simulink model "Chapter_4_Section_3_Model"  (R2017a)
settings: Solver=ode4  StartTime=0.0  StopTime=200  FixedStep=stp_sz  MaxStep=.0001  MinStep=.00005  RelTol=1e-7  AbsTol=1e-7  EnableMultiTasking=on
InitFcn:
  | load Chapter_4_Section_3
  | warning off
StopFcn:
  | save data.mat u_simulation v_simulation psi_simulation r_simulation npr_user_provided npr_achievable alpha_user_provided alpha_achievable stp_sz
  | clear all
  | load('data.mat')
  | delete('data.mat')
values from neighbouring files (symbols this model uses):
  A_disk = 13.2025431267    [Chapter_4_Section_3.mat]
  a_r11 = [-0.000865667853776 -0.901318756108 0.00874486630837 -0.00765974060328 0.00955717632387 0.00641813989061 -0.011076069832 0.00201248118094 -0.00501952733262 0.00315605586996 -0.00210851076531 0.0148609220099 ... (324 elements, 18x18)]    [Chapter_4_Section_3.mat]
  a_r13 = [-0.0294995912119 -4.91037219533 -0.00332739568397 0.0888755061346 -0.00681796875441 0.183812407485 0.0112008036726 0.10429312155 -0.0251601482875 -0.228675692165 0.00453476042855 0.0594697753606 ... (169 elements, 13x13)]    [Chapter_4_Section_3.mat]
  a_r15 = [-0.00127786555898 0.776225741104 -0.00474776997752 -0.00131066749835 0.0137520402687 -0.00211384579247 8.8019955143e-05 -0.00028996241197 -0.00129826872567 -0.0202543144732 0.0030370404199 -0.00453425604591 ... (169 elements, 13x13)]    [Chapter_4_Section_3.mat]
  a_r22 = [-0.000797108949019 -1.01015556887 0.00406573750109 -0.00111578544774 0.00423859757219 -0.00799128279013 0.00569024815652 -0.0167562674532 0.00334935655618 -0.000712432292804 0.00154242142086 0.00240437743229 ... (169 elements, 13x13)]    [Chapter_4_Section_3.mat]
  a_r24 = [-0.000686927823555 -0.95665602689 0.00244839898375 0.00145613314595 -0.00607023426216 0.0163996841317 0.00152022458075 -0.000736874734971 -0.00294919321651 -0.000761800577268 -0.00251686123035 -0.00197732815976 ... (169 elements, 13x13)]    [Chapter_4_Section_3.mat]
  a_r26 = [-0.194397873228 1.89810259721 -0.0873186628061 -0.241231729519 0.281206161775 -0.16994038615 -0.116565511469 -0.0496572593209 0.0216084469732 0.0912933167406 0.0299797727001 0.0314987707028 ... (169 elements, 13x13)]    [Chapter_4_Section_3.mat]
  a_r31 = [-0.00489112559449 -3.89960530455 -0.0361162658575 0.0265931197764 0.0034376033088 0.000316401308368 -0.0243996243526 0.0792200139858 -0.023187698537 -0.0726743997029 0.00400632061963 -0.0350516560041 ... (169 elements, 13x13)]    [Chapter_4_Section_3.mat]
  a_r33 = [-0.601431448276 0.50360246711 0.500115950342 -0.0452293844892 -0.0181314142185 -0.0323524621531 0.0355826051968 0.0329239610677 0.0940919952313 0.0566642992805 -0.0379178935102 0.0254835488846 ... (169 elements, 13x13)]    [Chapter_4_Section_3.mat]
  a_r35 = [-0.861988746714 -0.582511154549 0.34264856173 -0.0655310417272 -0.417167685168 0.183176698588 -0.473887691644 -0.225677727522 -0.133571139717 -0.218168843707 0.0850592077583 -0.0257492082836 ... (169 elements, 13x13)]    [Chapter_4_Section_3.mat]
  a_r42 = [-0.000411079312172 -0.966350953459 0.00419936729713 0.00358740198521 -0.00356571428733 -0.00958951498266 -0.00230062261745 -3.48708248632e-05 -0.00350313209064 -0.00772126326768 -0.0011918234528 -0.00149424537901 ... (169 elements, 13x13)]    [Chapter_4_Section_3.mat]
  a_r44 = [-0.000156115728087 -0.944139704333 -0.00242185567679 0.00620214191605 0.00232565005277 -0.00625050722164 0.00126021167241 -0.000681873506535 0.0011931592381 -0.00289361611357 -0.00138182415247 -0.00252837386868 ... (169 elements, 13x13)]    [Chapter_4_Section_3.mat]
  a_r46 = [-0.000218462457517 1.89677852742 0.00896242354968 -0.00290259500747 0.00225128874867 0.00254539590487 0.00120681433209 0.00261900930035 0.00149629742842 0.000796832004109 0.00199591847947 0.00352664402036 ... (169 elements, 13x13)]    [Chapter_4_Section_3.mat]
  a_r51 = [-0.0010898880101 0.776080724329 0.000225388678941 0.00375234840616 -0.00838297691459 -0.00447310416982 -0.0119510882322 -0.00692765468718 0.00227273345413 -0.0063592610709 0.000914007544175 0.00943534814934 ... (169 elements, 13x13)]    [Chapter_4_Section_3.mat]
  a_r53 = [-0.83377539904 0.569677058563 0.434285019976 0.157205409215 -0.397195569542 -0.255164078245 -0.141246880777 0.177451291189 -0.182828550566 0.0648162508754 0.244251292681 0.160100487197 ... (169 elements, 13x13)]    [Chapter_4_Section_3.mat]
  a_r55 = [-0.000352406331634 0.764343029796 0.00339830320259 -0.000678251137483 -0.00243783779313 -0.00215979913278 0.00196909451093 -0.00577428819561 -0.00349811892924 -0.00488920883323 0.00112064970343 0.000774855197444 ... (169 elements, 13x13)]    [Chapter_4_Section_3.mat]
  a_r62 = [-0.546519039316 -1.22303009993 0.393735845548 -0.120016588191 0.38151861373 -0.213578592342 -0.602267954372 -0.105716444149 -0.153151371839 -0.163939447448 -0.555540353196 0.0685401630267 ... (169 elements, 13x13)]    [Chapter_4_Section_3.mat]
  a_r64 = [-0.0406191100017 -5.18251105957 -0.115497941507 -0.0935821370219 0.180972853448 -0.0201998949456 -0.0698170640352 -0.0736823539521 -0.034828919888 0.0876659960431 -0.0419335596239 -0.0240984963396 ... (169 elements, 13x13)]    [Chapter_4_Section_3.mat]
  a_r66 = [-0.00276803466684 1.11530008029 0.0229779449181 0.0262185319857 0.00628472844795 0.000156167369042 -0.00250093023805 -0.0114435042874 -0.00826774415326 -0.00991601759993 -0.00812142854996 0.0148245002111 ... (169 elements, 13x13)]    [Chapter_4_Section_3.mat]
  A_rudder = 6    [Chapter_4_Section_3.mat]
  alpha_max = 0.392699081699    [Chapter_4_Section_3.mat]
  b_r11 = [-1.91804272115 -67.7547902158 12.3212653748 -6.25011871643 13.082442224 5.48501776184 -10.1596546398 2.56004852009 -4.74360113798 3.95981895348 -2.02856412397 18.3264246889 ... (18 elements, 18x1)]    [Chapter_4_Section_3.mat]
  b_r13 = [9.68113335046 8.54720242819 0.883931047444 -5.56576078332 1.72641800243 -13.8756826027 -2.702777864 -9.4621991361 5.92943514782 22.6516835054 -1.0074598861 -6.31102592982 ... (13 elements, 13x1)]    [Chapter_4_Section_3.mat]
  b_r22 = [-8.230214728 -263.156134326 24.2327808151 -4.87921448873 19.1715641288 -45.8768653263 26.6325387064 -91.9399975548 16.6663243552 -3.80929112747 7.68030110892 12.8381492859 ... (13 elements, 13x1)]    [Chapter_4_Section_3.mat]
  b_r24 = [20.6689502907 674.321335078 -41.3637763247 -19.2444203625 82.0775505272 -259.897803047 -22.2545830602 11.3827604156 43.2189922355 11.7516897475 36.9394390446 30.4503929007 ... (13 elements, 13x1)]    [Chapter_4_Section_3.mat]
  b_r26 = [206.794755218 -62.242559329 24.5666904254 184.158146246 -103.419961827 115.160111337 76.4499795128 20.3457431208 -13.1704465249 -41.5730935141 -18.1334448714 -14.4641153742 ... (13 elements, 13x1)]    [Chapter_4_Section_3.mat]
  b_r31 = [3.76230189948 5.16928151238 2.64945725635 -18.4251953385 -2.0625905672 -0.18887543415 4.20433084471 -14.07893046 13.0563354882 16.4007691754 -2.13849071942 8.28528512456 ... (13 elements, 13x1)]    [Chapter_4_Section_3.mat]
  b_r33 = [-425.265727934 16.4952177922 163.76327445 -15.539902078 -6.59006558263 -11.1862310226 12.8543123126 11.4260264426 33.8206936715 19.7626944669 -13.5783728882 8.91023495161 ... (13 elements, 13x1)]    [Chapter_4_Section_3.mat]
  b_r35 = [955.467057384 23.8174564739 -126.402446683 48.3788727465 168.435579445 -128.161344325 216.24493699 142.979450788 65.1193355403 134.911935543 -50.7648858119 13.1799100865 ... (13 elements, 13x1)]    [Chapter_4_Section_3.mat]
  b_r42 = [15.9360311823 665.959154186 -98.5777560157 -55.5400651809 61.9220987195 200.312325561 47.5124103398 0.631683490985 64.1219861023 155.750535985 22.3985447876 29.803792586 ... (13 elements, 13x1)]    [Chapter_4_Section_3.mat]
  b_r44 = [-27.1891200017 -1761.50772747 -283.391471232 367.311489951 182.522124626 -579.755911925 104.353356772 -62.2376848714 99.3185259533 -260.784153955 -116.536414334 -226.454300618 ... (13 elements, 13x1)]    [Chapter_4_Section_3.mat]
  b_r46 = [-26.6906838426 431.487773123 657.709356633 -144.976364483 114.646575538 180.775978583 85.0953284375 135.592940904 78.9082960716 55.2973047721 106.740201988 241.432567993 ... (13 elements, 13x1)]    [Chapter_4_Section_3.mat]
  b_r51 = [-27.9768378982 741.05041888 2.33758926296 57.3995096963 -127.005620965 -47.2947833409 -133.876425682 -98.5907202753 26.0445243962 -88.3721242204 10.7680008324 130.122749963 ... (13 elements, 13x1)]    [Chapter_4_Section_3.mat]
  b_r53 = [949.455593416 -23.2452293814 -157.318364745 -121.412853107 173.067821874 177.10214052 64.7164189373 -120.452255472 86.0623964314 -43.0643550932 -116.39314584 -105.497696438 ... (13 elements, 13x1)]    [Chapter_4_Section_3.mat]
  b_r55 = [-217.127382907 9506.32343029 1148.82922273 -188.742556573 -694.43970838 -709.996440288 566.872400877 -1877.38940059 -1026.37679575 -1566.80129668 332.089563592 247.692614281 ... (13 elements, 13x1)]    [Chapter_4_Section_3.mat]
  b_r62 = [259.61149635 16.5485296799 -38.0095496792 45.1883806678 -40.3107166739 78.3455844965 73.5107367495 37.0054960802 51.6709447748 22.7410486275 84.4875008959 -21.9559289205 ... (13 elements, 13x1)]    [Chapter_4_Section_3.mat]
  b_r64 = [156.539833252 187.686482031 376.820920142 59.4312894666 -548.902692032 17.0176436095 70.7484878223 206.821047291 37.1716677759 -243.032149857 114.824775027 27.0037475025 ... (13 elements, 13x1)]    [Chapter_4_Section_3.mat]
  b_r66 = [-314.266256408 5285.46587095 1093.01941502 1627.30071258 387.633965073 8.0986510694 -130.443621448 -701.343286032 -436.49966457 -600.0481003 -433.735518303 884.367320612 ... (13 elements, 13x1)]    [Chapter_4_Section_3.mat]
  bettas_CQ = [0 5.39 17.77 34.97 50.79 58.7 64.55 68.33 73.49 85.2 93.11 102.75 ... (40 elements, 1x40)]    [Chapter_4_Section_3.mat]    (also in looking_up_n.m = [0 5.39 17.77 34.97 50.79 58.7 64.55 68.33 73.49 85.2 93.11 )
  bettas_CT = [0 5.37 16.73 33.6 44.63 60.82 73.22 80.46 86.3 92.15 100.41 110.74 ... (52 elements, 1x52)]    [Chapter_4_Section_3.mat]    (also in looking_up_n.m = [0 5.37 16.73 33.6 44.63 60.82 73.22 80.46 86.3 92.15 100.41)
  c_r11 = [1.91804272142 -67.7547902158 -12.3212653748 -6.25011871643 -13.082442224 5.48501776185 -10.1596546398 -2.56004852009 -4.74360113798 -3.95981895348 -2.02856412396 -18.3264246889 ... (18 elements, 1x18)]    [Chapter_4_Section_3.mat]
  c_r13 = [9.68113335045 -8.54720242824 0.883931047418 5.56576078332 1.72641800244 13.8756826027 -2.702777864 9.4621991361 5.92943514781 -22.6516835054 -1.0074598861 6.31102592982 ... (13 elements, 1x13)]    [Chapter_4_Section_3.mat]
  c_r22 = [8.23021472807 -263.156134326 -24.2327808151 -4.87921448871 19.1715641288 45.8768653263 26.6325387064 91.9399975548 16.6663243552 3.80929112749 7.68030110892 -12.8381492859 ... (13 elements, 1x13)]    [Chapter_4_Section_3.mat]
  c_r24 = [20.6689502903 -674.321335078 -41.3637763247 19.2444203625 -82.0775505271 -259.897803047 22.2545830602 11.3827604156 -43.2189922355 11.7516897475 -36.9394390446 30.4503929007 ... (13 elements, 1x13)]    [Chapter_4_Section_3.mat]
  c_r26 = [-206.794755218 -62.2425593289 24.5666904254 -184.158146246 -103.419961827 -115.160111337 -76.4499795128 20.3457431209 13.1704465249 -41.5730935141 18.1334448714 -14.4641153742 ... (13 elements, 1x13)]    [Chapter_4_Section_3.mat]
  c_r31 = [3.76230189951 -5.16928151238 -2.64945725636 -18.4251953385 -2.0625905672 -0.188875434257 -4.2043308447 14.07893046 13.0563354882 -16.4007691754 -2.13849071943 -8.28528512456 ... (13 elements, 1x13)]    [Chapter_4_Section_3.mat]
  c_r33 = [-425.265727934 -16.4952177923 -163.76327445 15.539902078 -6.5900655826 11.1862310226 12.8543123126 -11.4260264426 33.8206936715 -19.7626944669 -13.5783728882 -8.91023495161 ... (13 elements, 1x13)]    [Chapter_4_Section_3.mat]
  c_r35 = [-955.467057384 23.8174564746 -126.402446683 -48.3788727464 168.435579445 128.161344325 216.24493699 -142.979450788 65.1193355403 -134.911935543 50.7648858119 13.1799100865 ... (13 elements, 1x13)]    [Chapter_4_Section_3.mat]
  c_r42 = [15.9360311824 -665.959154186 -98.5777560157 55.5400651809 -61.9220987195 200.312325561 47.5124103398 -0.631683490192 -64.1219861023 155.750535985 -22.3985447876 29.803792586 ... (13 elements, 1x13)]    [Chapter_4_Section_3.mat]
  c_r44 = [27.189120009 -1761.50772747 283.391471232 367.311489951 182.522124626 579.755911925 104.353356772 62.2376848713 99.3185259533 260.784153955 -116.536414334 226.454300618 ... (13 elements, 1x13)]    [Chapter_4_Section_3.mat]
  c_r46 = [26.6906838375 431.487773123 -657.709356633 -144.976364484 114.646575538 -180.775978583 -85.0953284373 135.592940904 78.9082960717 -55.297304772 106.740201988 -241.432567993 ... (13 elements, 1x13)]    [Chapter_4_Section_3.mat]
  c_r51 = [27.9768378982 741.05041888 2.33758926325 -57.3995096963 127.005620965 -47.2947833409 -133.876425682 98.5907202753 26.0445243962 88.3721242204 10.7680008324 -130.122749963 ... (13 elements, 1x13)]    [Chapter_4_Section_3.mat]
  c_r53 = [-949.455593416 -23.2452293814 -157.318364745 121.412853107 173.067821874 -177.10214052 64.7164189374 120.452255472 86.0623964314 43.0643550932 -116.39314584 105.497696438 ... (13 elements, 1x13)]    [Chapter_4_Section_3.mat]
  c_r55 = [217.12738291 9506.32343029 -1148.82922273 -188.742556576 -694.43970838 709.996440288 566.872400876 1877.38940059 -1026.37679575 1566.80129668 332.089563594 -247.69261428 ... (13 elements, 1x13)]    [Chapter_4_Section_3.mat]
  c_r62 = [-259.61149635 16.5485296799 -38.0095496792 -45.1883806678 -40.3107166739 -78.3455844965 73.5107367495 -37.0054960802 -51.6709447748 22.7410486275 84.4875008959 21.9559289205 ... (13 elements, 1x13)]    [Chapter_4_Section_3.mat]
  c_r64 = [-156.539833251 187.686482031 -376.820920142 59.4312894666 548.902692032 17.0176436097 70.7484878223 -206.82104729 37.1716677758 243.032149857 -114.824775027 27.0037475025 ... (13 elements, 1x13)]    [Chapter_4_Section_3.mat]
  c_r66 = [314.266256408 5285.46587095 1093.01941502 -1627.30071258 -387.633965073 8.09865107118 -130.443621448 701.343286032 -436.49966457 600.0481003 -433.735518303 -884.367320612 ... (13 elements, 1x13)]    [Chapter_4_Section_3.mat]
  CQs = [0.008 0.007 -0.002 -0.018 -0.037 -0.049 -0.06 -0.065 -0.068 -0.059 -0.057 -0.059 ... (40 elements, 1x40)]    [Chapter_4_Section_3.mat]    (also in looking_up_n.m = -0.1.*[-0.08 -0.07 0.02 0.18 0.37 0.49 0.6 0.65 0.68 0.59 0.)
  CTs = [0.32 0.29 0.19 0.01 -0.16 -0.46 -0.7 -0.77 -0.7 -0.63 -0.63 -0.69 ... (52 elements, 1x52)]    [Chapter_4_Section_3.mat]    (also in looking_up_n.m = [0.32 0.29 0.19 0.01 -0.16 -0.46 -0.7 -0.77 -0.7 -0.63 -0.63)
  d_r11 = 95.5285227708    [Chapter_4_Section_3.mat]
  d_r13 = -14.1628545989    [Chapter_4_Section_3.mat]
  d_r22 = 1468.51041279    [Chapter_4_Section_3.mat]
  d_r24 = -9785.77027698    [Chapter_4_Section_3.mat]
  d_r26 = -1700.92421833    [Chapter_4_Section_3.mat]
  d_r31 = -0.95522945761    [Chapter_4_Section_3.mat]
  d_r33 = 3827.81220596    [Chapter_4_Section_3.mat]
  d_r35 = -19539.5268707    [Chapter_4_Section_3.mat]
  d_r42 = -9418.04264727    [Chapter_4_Section_3.mat]
  d_r44 = 68252.1479072    [Chapter_4_Section_3.mat]
  d_r46 = -10162.1377852    [Chapter_4_Section_3.mat]
  d_r51 = 12054.4514237    [Chapter_4_Section_3.mat]
  d_r53 = -19539.5038011    [Chapter_4_Section_3.mat]
  d_r55 = 1991036.95813    [Chapter_4_Section_3.mat]
  d_r62 = -1405.47636444    [Chapter_4_Section_3.mat]
  d_r64 = -12342.2523681    [Chapter_4_Section_3.mat]
  d_r66 = 610786.440495    [Chapter_4_Section_3.mat]
  DEN = 5.34671106464e+28    [Chapter_4_Section_3.mat]
  dist_LOS = [-50 -49 -48 -47 -46 -45 -44 -43 -42 -41 -40 -39 ... (1051 elements, 1x1051)]    [Chapter_4_Section_3.mat]
  Dpr = 4.1    [Chapter_4_Section_3.mat]    (also in looking_up_n.m = u(4))
  Dw = 0.110526315789    [Chapter_4_Section_3.mat]
  dx = 10    [Chapter_4_Section_3.mat]
  dxr = 48.75    [Chapter_4_Section_3.mat]
  dy = 2    [Chapter_4_Section_3.mat]
  dz = 0.8    [Chapter_4_Section_3.mat]
  dzr = 0.514285714286    [Chapter_4_Section_3.mat]
  g = 10    [Chapter_4_Section_3.mat]
  gravity = 10    [Chapter_4_Section_3.mat]
  INDEX = [1 2 3 4 5 6 7 8 9]    [Chapter_4_Section_3.mat]
  Ix = 724554000    [Chapter_4_Section_3.mat]
  Iy = 4528460000    [Chapter_4_Section_3.mat]
  Iz = 4528460000    [Chapter_4_Section_3.mat]
  k_wave = [0.0157865285852 0.0224311321394 0.0345394916241 0.0578593033576 0.0778685019714 0.0983501894009 0.10403521245 0.134043066308 0.155236404606 0.203205074918 0.220032771713 0.262178651673 ... (20 elements, 1x20)]    [Chapter_4_Section_3.mat]
  Last_Pt_Accuracy = 30    [Chapter_4_Section_3.mat]
  LBP = 100    [Chapter_4_Section_3.mat]
  m = 7264000    [Chapter_4_Section_3.mat]
  phase = [4.61787442739 6.09845039199 5.44708367148 0.54182753101 2.30238916367 2.31974450279 4.30416083443 3.75697809799 4.95971993271 2.31003141527 1.29451121971 0.54454197722 ... (20 elements, 1x20)]    [Chapter_4_Section_3.mat]
  phi_0 = 0    [Chapter_4_Section_3.mat]
  psi_0 = 0    [Chapter_4_Section_3.mat]
  R_convrg = 220    [Chapter_4_Section_3.mat]
  radius_LOS = [166.575605377 166.637026665 166.698699321 166.760625342 166.82280675 166.885245588 166.947943925 167.010903854 167.074127493 167.137616985 167.201374499 167.265402228 ... (1051 elements, 1x1051)]    [Chapter_4_Section_3.mat]
  raw = 1000    [Chapter_4_Section_3.mat]    (also in looking_up_n.m = u(3))
  s = 0.15    [Chapter_4_Section_3.mat]
  S11 = 5.22457985714e+28    [Chapter_4_Section_3.mat]
  S13 = 3.79917831589e+26    [Chapter_4_Section_3.mat]
  S15 = -4.97006200608e+19    [Chapter_4_Section_3.mat]
  S22 = 4.58630932583e+28    [Chapter_4_Section_3.mat]
  S24 = 9.38800137353e+19    [Chapter_4_Section_3.mat]
  S26 = 1.30387886946e+18    [Chapter_4_Section_3.mat]
  S31 = 3.83422033136e+26    [Chapter_4_Section_3.mat]
  S33 = 1.77296018417e+28    [Chapter_4_Section_3.mat]
  S35 = 2.44593333777e+19    [Chapter_4_Section_3.mat]
  S42 = 8.93369784557e+19    [Chapter_4_Section_3.mat]
  S44 = 7.37931315974e+19    [Chapter_4_Section_3.mat]
  S46 = 27990784014.6    [Chapter_4_Section_3.mat]
  S51 = -4.98658939538e+19    [Chapter_4_Section_3.mat]
  S53 = 2.45188465874e+19    [Chapter_4_Section_3.mat]
  S55 = 1.18069051188e+19    [Chapter_4_Section_3.mat]
  S62 = 1.30580221388e+18    [Chapter_4_Section_3.mat]
  S64 = 23535167243.9    [Chapter_4_Section_3.mat]
  S66 = 1.18069078235e+19    [Chapter_4_Section_3.mat]
  ... (+18 more)
undefined symbols (not defined in the file or in its folder): magnitude
libraries: simulink x9
(part 2 of 6)

== system Chapter_4_Section_3_Model/Ship_Model/Ship Dynamics with Environmental Forces and Memory Effect/Linear Damping ==
  In1 : Inport
  In2 : Inport  Port=2
  In3 : Inport  Port=3
  In4 : Inport  Port=4
  In5 : Inport  Port=5
  In6 : Inport  Port=6
  Constant1 : Constant
  Constant{2,4,7,11} (4 alike) : Constant  Value=8
  Constant14 : Constant
  Constant16 : Constant  Value=Iz
  Constant20 : Constant  Value=m
  Constant22 : Constant  Value=m
  Constant28 : Constant  Value=m
  Constant3 : Constant  Value=Ix
  Constant6 : Constant  Value=Iy
  Gain : Gain  Gain=-1
  Mux : Mux  Inputs=6
  Product{2..5,7..8} (6 alike) : Product  Inputs=3  RndMeth=Zero
  Out1 : Outport
  wires:
  Constant28/1 -> Product5/2
  Constant2/1 -> Product5/3
  Mux/1 -> Gain/1
  Constant3/1 -> Product2/2
  Constant4/1 -> Product2/3
  Constant6/1 -> Product3/2
  Constant7/1 -> Product3/3
  Constant16/1 -> Product4/2
  Constant11/1 -> Product4/3
  Gain/1 -> Out1/1
  Product5/1 -> Mux/3
  Product2/1 -> Mux/4
  Product3/1 -> Mux/5
  Constant20/1 -> Product7/2
  Constant1/1 -> Product7/3
  Constant22/1 -> Product8/2
  Constant14/1 -> Product8/3
  Product7/1 -> Mux/1
  Product8/1 -> Mux/2
  Product4/1 -> Mux/6
  In1/1 -> Product7/1
  In2/1 -> Product8/1
  In3/1 -> Product5/1
  In4/1 -> Product2/1
  In5/1 -> Product3/1
  In6/1 -> Product4/1

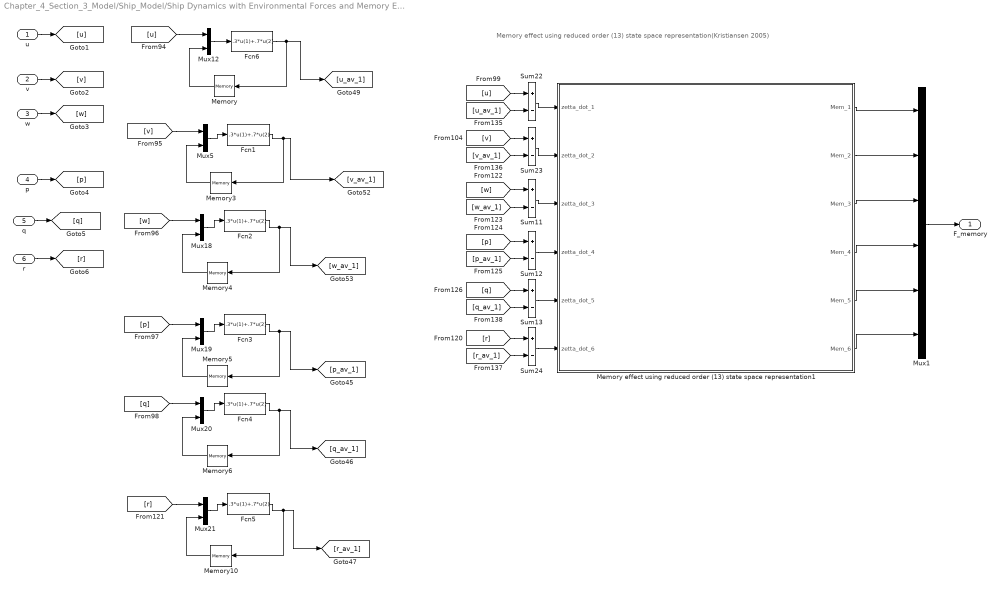
== system Chapter_4_Section_3_Model/Ship_Model/Ship Dynamics with Environmental Forces and Memory Effect/Memory effect using reduced order (13) state space representation(Kristiansen 2005) ==
  note: Memory effect using reduced order (13) state space representation(Kristiansen 2005)
  u : Inport
  v : Inport  Port=2
  w : Inport  Port=3
  p : Inport  Port=4
  q : Inport  Port=5
  r : Inport  Port=6
  Fcn{1..6} (6 alike) : Fcn  Expr=.3*u(1)+.7*u(2)
  Memory{,3..6,10} (6 alike) : Memory  InheritSampleTime=on
  Memory effect using reduced order (13) state space representation1 : Subsystem
  Mux1 : Mux  Inputs=6
  Mux{5,12,18..21} (6 alike) : Mux  Inputs=2
  Sum{11..13,22..24} (6 alike) : Sum  Inputs=+-
  F_memory : Outport
  wires:
  Memory effect using reduced order (13) state space representation1/1(Mem_1) -> Mux1/1
  Memory effect using reduced order (13) state space representation1/2(Mem_2) -> Mux1/2
  Memory effect using reduced order (13) state space representation1/3(Mem_3) -> Mux1/3
  Memory effect using reduced order (13) state space representation1/4(Mem_4) -> Mux1/4
  Memory effect using reduced order (13) state space representation1/5(Mem_5) -> Mux1/5
  Memory effect using reduced order (13) state space representation1/6(Mem_6) -> Mux1/6
  Mux1/1 -> F_memory/1
  Memory/1 -> Mux12/2
  Mux12/1 -> Fcn6/1
  [u] -> Mux12/1
  Fcn6/1 -> Memory/1, [u_av_1]
  Memory3/1 -> Mux5/2
  Mux5/1 -> Fcn1/1
  [v] -> Mux5/1
  Fcn1/1 -> Memory3/1, [v_av_1]
  Memory4/1 -> Mux18/2
  Mux18/1 -> Fcn2/1
  [w] -> Mux18/1
  Fcn2/1 -> Memory4/1, [w_av_1]
  Memory5/1 -> Mux19/2
  Mux19/1 -> Fcn3/1
  [p] -> Mux19/1
  Fcn3/1 -> Memory5/1, [p_av_1]
  Memory6/1 -> Mux20/2
  Mux20/1 -> Fcn4/1
  [q] -> Mux20/1
  Fcn4/1 -> Memory6/1, [q_av_1]
  Memory10/1 -> Mux21/2
  Mux21/1 -> Fcn5/1
  [r] -> Mux21/1
  Fcn5/1 -> Memory10/1, [r_av_1]
  Sum23/1 -> Memory effect using reduced order (13) state space representation1/2(zetta_dot_2)
  Sum24/1 -> Memory effect using reduced order (13) state space representation1/6(zetta_dot_6)
  [u] -> Sum22/1
  [u_av_1] -> Sum22/2
  Sum22/1 -> Memory effect using reduced order (13) state space representation1/1(zetta_dot_1)
  [v] -> Sum23/1
  [v_av_1] -> Sum23/2
  [r] -> Sum24/1
  [r_av_1] -> Sum24/2
  [w] -> Sum11/1
  [w_av_1] -> Sum11/2
  [p] -> Sum12/1
  [p_av_1] -> Sum12/2
  [q] -> Sum13/1
  [q_av_1] -> Sum13/2
  Sum11/1 -> Memory effect using reduced order (13) state space representation1/3(zetta_dot_3)
  Sum12/1 -> Memory effect using reduced order (13) state space representation1/4(zetta_dot_4)
  Sum13/1 -> Memory effect using reduced order (13) state space representation1/5(zetta_dot_5)
  u/1 -> [u]
  v/1 -> [v]
  w/1 -> [w]
  p/1 -> [p]
  q/1 -> [q]
  r/1 -> [r]

== system Chapter_4_Section_3_Model/Ship_Model/Ship Dynamics with Environmental Forces and Memory Effect/Rudder ==
  note: Rudder Forces based on  Lift and Drag coefficients (CL and CD)
      | of symmetrical NACA wing sections for t=0.06 and AR=29
  note: Lift and drag forces of the rudder
  note: checking if the flow is hitting the rudder from the front (u>0)
      | or from the back (u<0)
  Fth_next_step : Inport
  u : Inport  Port=2
  v : Inport  Port=3
  alpha in : Inport  Port=4
  Abs : Abs
  Constant6 : Constant
  Fcn : Fcn  Expr=2*u(1)/(raw*A_disk)+u(2)^2
  Fcn2 : Fcn  Expr=sqrt(u(1)^2+u(2)^2)
  Math Function : Math  Operator=sqrt  SaturateOnIntegerOverflow=on
  Memory1 : Memory  InheritSampleTime=on
  Mux : Mux  Inputs=2
  Mux2 : Mux  Inputs=2
  Product1 : Product  RndMeth=Zero
  Rudder Dynamics : Subsystem
  Sum3 : Sum  Inputs=|+|-|
  Trigonometric Function : Trigonometry  Operator=atan2
  minus : Gain  Gain=-1
  wake factor1 : Constant  Value=w
  Fr_x : Outport
  Fr_y : Outport  Port=2
  Fr_rudder : Outport  Port=3
  alpha_e : Outport  Port=4
  V : Outport  Port=5
  wires:
  [V] -> Rudder Dynamics/1(V)
  Fth_next_step/1 -> [Fth_next_step]
  Mux/1 -> Fcn/1
  [Fth_next_step] -> Mux/1
  Constant6/1 -> Sum3/1
  wake factor1/1 -> Sum3/2
  Abs/1 -> Math Function/1
  Fcn/1 -> Abs/1
  Math Function/1 -> [Vrudder], V/1
  v/1 -> [v]
  u/1 -> Product1/1
  Sum3/1 -> Product1/2
  Product1/1 -> [Vpr]
  [Vpr] -> Mux/2
  [v] -> Mux2/2
  [v] -> minus/1
  Trigonometric Function/1 -> alpha_e/1, [alpha_e]
  Rudder Dynamics/1(Fr_x) -> Fr_x/1
  Rudder Dynamics/2(Fr_y) -> Fr_y/1
  [Vrudder] -> Mux2/1
  Mux2/1 -> Fcn2/1
  Fcn2/1 -> [V]
  minus/1 -> Trigonometric Function/1
  [Vrudder] -> Trigonometric Function/2
  [alpha] -> Rudder Dynamics/2(alpha)
  Memory1/1 -> Rudder Dynamics/3(alpha_e)
  [alpha_e] -> Memory1/1
  alpha in/1 -> [alpha]
  Rudder Dynamics/3(Frudder) -> Fr_rudder/1

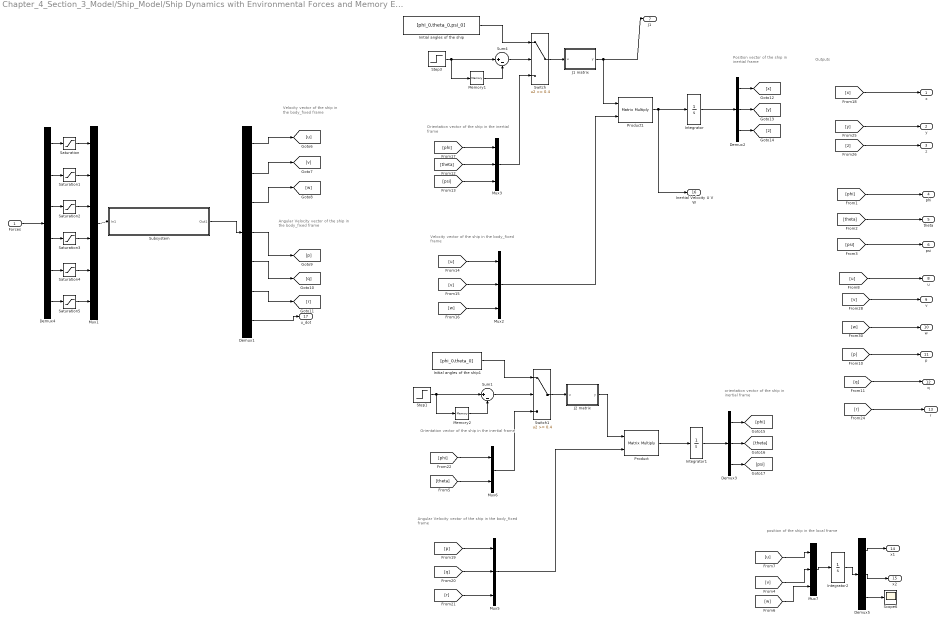
== system Chapter_4_Section_3_Model/Ship_Model/Ship Dynamics with Environmental Forces and Memory Effect/Six DOF State Integrator of the Ship ==
  note: Position vector
      | of the ship in
      |  inertial frame
  note: Orientation vector of the ship in the
      |  inertial frame
  note: orientation vector
      | of the ship in
      |  inertial frame
  note: Orientation vector of the ship in the
      |  inertial frame
  note: Velocity vector of the ship in the
      | body_fixed frame
  note: Angular Velocity  vector of the ship in the
      | body_fixed frame
  note: Outputs
  note: position of the ship in the local frame
  note: Velocity vector
      | of the ship in
      | the body_fixed frame
  note: Angular Velocity
      |  vector of the
      |  ship in the
      | body_fixed frame
  Forces : Inport
  Demux1 : Demux  Outputs=7
  Demux2 : Demux  Outputs=3
  Demux3 : Demux  Outputs=3
  Demux4 : Demux  Outputs=6
  Demux5 : Demux  Outputs=3
  Initial angles of the ship : Constant  Value=[phi_0,theta_0,psi_0]
  Initial angles of the ship1 : Constant  Value=[phi_0,theta_0]
  Integrator : Integrator  InitialCondition=[x0,y0,z0]
  Integrator1 : Integrator  InitialCondition=[phi_0,theta_0,psi_0]
  Integrator2 : Integrator  InitialCondition=[x0,y0,z0]
  J1 matrix : MATLAB Function  TreatAsAtomicUnit=on
  J2 matrix : MATLAB Function  TreatAsAtomicUnit=on
  Memory1 : Memory  InheritSampleTime=on
  Memory2 : Memory  InheritSampleTime=on
  Mux1 : Mux  Inputs=6
  Mux{2..3,5,7} (4 alike) : Mux  Inputs=3
  Mux6 : Mux  Inputs=2
  Product : Product  Multiplication=Matrix(*)  RndMeth=Zero
  Product1 : Product  Multiplication=Matrix(*)  RndMeth=Zero
  Saturation{,2..5} (5 alike) : Saturate  UpperLimit=1e9  LowerLimit=-1e9
  Saturation1 : Saturate  UpperLimit=1e8  LowerLimit=-1e8
  Scope6 : Scope
  Step1 : Step  Time=0  SampleTime=0
  Step3 : Step  Time=0  SampleTime=0
  Subsystem : Subsystem
  Sum1 : Sum  Inputs=|+-
  Sum4 : Sum  Inputs=|+-
  Switch : Switch  Threshold=0.4
  Switch1 : Switch  Threshold=0.4
  x : Outport
  y : Outport  Port=2
  z : Outport  Port=3
  phi : Outport  Port=4
  theta : Outport  Port=5
  psi : Outport  Port=6
  J1 : Outport  Port=7
  u : Outport  Port=8
  v : Outport  Port=9
  w : Outport  Port=10
  p : Outport  Port=11
  q : Outport  Port=12
  r : Outport  Port=13
  x1 : Outport  Port=14
  x2 : Outport  Port=15
  Inertial Velcoity U V W : Outport  Port=16
  u_dot : Outport  Port=17
  wires:
  Product1/1 -> Integrator/1, Inertial Velcoity U V W/1
  Integrator/1 -> Demux2/1
  Demux2/1 -> [x]
  Demux2/2 -> [y]
  Demux2/3 -> [z]
  Initial angles of the ship/1 -> Switch/1
  [phi] -> Mux3/1
  [theta] -> Mux3/2
  [psi] -> Mux3/3
  Mux3/1 -> Switch/3
  Switch/1 -> J1 matrix/1(u)
  Integrator1/1 -> Demux3/1
  Demux3/1 -> [phi]
  Demux3/2 -> [theta]
  Demux3/3 -> [psi]
  Initial angles of the ship1/1 -> Switch1/1
  [phi] -> Mux6/1
  [theta] -> Mux6/2
  Mux6/1 -> Switch1/3
  Switch1/1 -> J2 matrix/1(u)
  Product/1 -> Integrator1/1
  [u] -> Mux2/1
  [v] -> Mux2/2
  [w] -> Mux2/3
  Mux2/1 -> Product1/2
  [p] -> Mux5/1
  [q] -> Mux5/2
  [r] -> Mux5/3
  J2 matrix/1(y) -> Product/1
  Mux5/1 -> Product/2
  J1 matrix/1(y) -> Product1/1, J1/1
  [x] -> x/1
  [y] -> y/1
  [z] -> z/1
  [phi] -> phi/1
  [theta] -> theta/1
  [psi] -> psi/1
  [u] -> u/1
  Step3/1 -> Memory1/1, Sum4/1
  Memory1/1 -> Sum4/2
  Sum4/1 -> Switch/2
  Step1/1 -> Memory2/1, Sum1/1
  Memory2/1 -> Sum1/2
  Sum1/1 -> Switch1/2
  [v] -> v/1
  [w] -> w/1
  [p] -> p/1
  [q] -> q/1
  [r] -> r/1
  Integrator2/1 -> Demux5/1
  Demux5/1 -> x1/1
  Demux5/2 -> x2/1
  Mux7/1 -> Integrator2/1
  [u] -> Mux7/1
  [v] -> Mux7/2
  [w] -> Mux7/3
  Demux5/3 -> Scope6/1
  Subsystem/1(Out1) -> Demux1/1
  Demux1/1 -> [u]
  Demux1/2 -> [v]
  Demux1/3 -> [w]
  Demux1/4 -> [p]
  Demux1/5 -> [q]
  Demux1/6 -> [r]
  Forces/1 -> Demux4/1
  Demux4/1 -> Saturation/1
  Demux4/2 -> Saturation1/1
  Demux4/3 -> Saturation2/1
  Demux4/4 -> Saturation3/1
  Saturation/1 -> Mux1/1
  Saturation1/1 -> Mux1/2
  Saturation2/1 -> Mux1/3
  Saturation3/1 -> Mux1/4
  Saturation4/1 -> Mux1/5
  Saturation5/1 -> Mux1/6
  Demux4/5 -> Saturation4/1
  Mux1/1 -> Subsystem/1(In1)
  Demux4/6 -> Saturation5/1
  Demux1/7 -> u_dot/1

== system Chapter_4_Section_3_Model/Ship_Model/Ship Dynamics with Environmental Forces and Memory Effect/Subsystem3 ==
  note: Propeller and Rudder Forces based on  Lift and Drag coefficients (CL and CD)
      | of symmetrical NACA wing sections for t=0.06 and AR=29
  note: Wageningen B4.70 ScrewPropeller with P/D=0.5
      |  (Ct and CQ Coefficients are taken from Kuiper 1992)
  note: comment: in case of the negative velocity of the ship (w.r.t its body fixed coordinates)
      | the velocity of flow enters the propeller from the back, with the velocity being u(because
      | the hull doesnt interact with the flow comming from the back).
  note: For very small amplitudes of thrust, it is considered to be identical to zero
  u : Inport
  npr : Inport  Port=2
  Abs : Abs
  Constant : Constant  Value=0
  Constant1 : Constant
  Constant2 : Constant  Value=0
  Mux8 : Mux  Inputs=6
  Product3 : Product  RndMeth=Zero
  Scope : Scope
  Scope1 : Scope
  Subsystem : Subsystem  TreatAsAtomicUnit=on
      settings: MinAlgLoopOccurrences=on
      mask Display: image(imread('propeller.jpg'))
  Sum2 : Sum  Inputs=|+|-|
  Switch : Switch
  Switch1 : Switch  Threshold=1
  Switch2 : Switch  Threshold=0.5
  initial control force in the sway{1..5} (5 alike) : Constant  Value=0
  wake factor : Constant  Value=w
  Fth_next_step : Outport
  Tpr_next_step : Outport  Port=2
  npr_next_step : Outport  Port=3
  F_thrust_vector : Outport  Port=4
  wires:
  u/1 -> [u]
  npr/1 -> [npr]
  Constant1/1 -> Sum2/1
  wake factor/1 -> Sum2/2
  Product3/1 -> Switch/1
  [Vpr] -> Subsystem/1(In1), Scope/1
  [npr] -> Scope1/1, Subsystem/2(In5)
  Subsystem/2(Out2) -> Tpr_next_step/1
  [u] -> Product3/2, Switch/2
  Sum2/1 -> Product3/1
  Switch/1 -> [Vpr]
  [u] -> Switch/3
  Subsystem/1(Out1) -> [Fth_next_step]
  [Fth_next_step] -> Abs/1, Switch1/1
  Constant2/1 -> Switch1/3
  Abs/1 -> Switch1/2
  Subsystem/3(Out3) -> npr_next_step/1
  initial control force in the sway2/1 -> Mux8/2
  initial control force in the sway3/1 -> Mux8/3
  initial control force in the sway1/1 -> Mux8/4
  initial control force in the sway4/1 -> Mux8/5
  initial control force in the sway5/1 -> Mux8/6
  Mux8/1 -> F_thrust_vector/1
  Constant/1 -> Switch2/1
  [First_time] -> Switch2/2
  Switch1/1 -> Switch2/3
  Switch2/1 -> Mux8/1, Fth_next_step/1

== system Chapter_4_Section_3_Model/Ship_Model/Ship Dynamics with Environmental Forces and Memory Effect/Wave Excitation Force ==
  x : Inport
  y : Inport  Port=2
  In3 : Inport  Port=3
  ksi : Inport  Port=4
  Constant9 : Constant  Value=2*pi
  Gain7 : Gain  Gain=180/pi
  Math Function1 : Math  Operator=mod  SaturateOnIntegerOverflow=on
  Sum7 : Sum  Inputs=|+|-|
  wave elevation from multiple frequencies2 : Subsystem
  F_wave_excitation_force : Outport
  wires:
  ksi/1 -> Sum7/1, wave elevation from multiple frequencies2/4(ksi)
  Gain7/1 -> wave elevation from multiple frequencies2/3(angle)
  Sum7/1 -> Math Function1/1
  Constant9/1 -> Math Function1/2
  Math Function1/1 -> Gain7/1
  wave elevation from multiple frequencies2/1(F) -> F_wave_excitation_force/1
  x/1 -> wave elevation from multiple frequencies2/1(X)
  y/1 -> wave elevation from multiple frequencies2/2(Y)
  In3/1 -> Sum7/2

== system Chapter_4_Section_3_Model/Ship_Model/Ship Dynamics with Environmental Forces and Memory Effect/Wind Force ==
  psi : Inport
  u : Inport  Port=2
  wind_angle_degree : Inport  Port=3
  velocity_wind : Inport  Port=4
  Constant1 : Constant  Value=2*pi
  Constant30 : Constant  Value=360
  Gain6 : Gain  Gain=180/pi
  Gain8 : Gain  Gain=pi/180
  Math Function1 : Math  Operator=mod  SaturateOnIntegerOverflow=on
  Math Function2 : Math  Operator=mod  SaturateOnIntegerOverflow=on
  Product6 : Product  RndMeth=Zero
  Sum4 : Sum  Inputs=|+|-|
  Sum5 : Sum  Inputs=|+|-|
  Trigonometric Function3 : Trigonometry  Operator=cos
  wind force : Subsystem
  F_wind : Outport
  wires:
  Constant30/1 -> Math Function2/2
  Gain6/1 -> Sum4/2
  Sum4/1 -> Math Function2/1
  Math Function2/1 -> [relative_wind_angle_deg]
  [relative_wind_angle_deg] -> Gain8/1
  Gain8/1 -> Trigonometric Function3/1
  Trigonometric Function3/1 -> Product6/2
  Sum5/1 -> wind force/2(relative velocity of the wind (m/s))
  [relative_wind_angle_deg] -> wind force/1(relative wind angle_degree)
  wind force/1(F_wind) -> F_wind/1
  Product6/1 -> Sum5/1
  u/1 -> Sum5/2
  wind_angle_degree/1 -> Sum4/1
  velocity_wind/1 -> Product6/1
  psi/1 -> Math Function1/1
  Math Function1/1 -> Gain6/1
  Constant1/1 -> Math Function1/2

== system Chapter_4_Section_3_Model/Ship_Model/LOS2/Breivik Model for psi/Heading Angle Filter ==
  In1 : Inport
  Transfer Fcn : TransferFcn  Numerator=[wn^2]  Denominator=[1 2*zeta*wn wn^2]
  Transfer Fcn1 : TransferFcn  Numerator=[wn]  Denominator=[1 wn]
  Transfer Fcn2 : TransferFcn  Numerator=[wn^2 0]  Denominator=[1 2*zeta*wn wn^2]
  Transfer Fcn3 : TransferFcn  Numerator=[wn^2 0 0]  Denominator=[1 2*zeta*wn wn^2]
  psi : Outport
  psi_dot : Outport  Port=2
  psi_dot_dot : Outport  Port=3
  wires:
  Transfer Fcn1/1 -> Transfer Fcn/1
  Transfer Fcn/1 -> psi/1, Transfer Fcn2/1, Transfer Fcn3/1
  In1/1 -> Transfer Fcn1/1
  Transfer Fcn2/1 -> psi_dot/1
  Transfer Fcn3/1 -> psi_dot_dot/1

== system Chapter_4_Section_3_Model/Ship_Model/LOS2/Breivik Model for psi/Subsystem2 ==
  note: x
  note: r
  x [-inf inf] : Inport
  Constant : Constant  Value=2*pi
  Gain : Gain  Gain=pi  SaturateOnIntegerOverflow=on  OutDataTypeStr=Inherit: Same as input  ParamDataTypeStr=Inherit: Same as input
  Math Function : Math  Operator=rem  SaturateOnIntegerOverflow=on
  Saturation : Saturate  UpperLimit=1e10  LowerLimit=-1e10
  Sign : Signum
  Sum : Sum  Inputs=|+-  SaturateOnIntegerOverflow=on
  Sum1 : Sum  Inputs=|++  SaturateOnIntegerOverflow=on
  y [-pi pi] : Outport
  wires:
  x [-inf inf]/1 -> Saturation/1
  Sign/1 -> Gain/1
  Gain/1 -> Sum/2, Sum1/2
  Sum1/1 -> Math Function/1
  Constant/1 -> Math Function/2
  Math Function/1 -> Sum/1
  Sum/1 -> y [-pi pi]/1
  Saturation/1 -> Sum1/1, Sign/1

== system Chapter_4_Section_3_Model/Ship_Model/LOS2/Breivik Model for psi/psi_d1 ==
  psi [-pi pi] : Inport
  Add : Sum
  Add1 : Sum
  Interval Test : simulink/Logic and Bit Operations/Interval Test  IntervalClosedRight=off  uplimit=0  IntervalClosedLeft=off  lowlimit=-pi  OutDataTypeStr=uint8
  Logical Operator : Logic  Operator=NOT  AllPortsSameDT=off  OutDataTypeStr=uint(8)
  Product : Product  RndMeth=Zero
  Product1 : Product  RndMeth=Zero
  angle1 : Constant  Value=2*pi
  psi [0 2pi] : Outport
  wires:
  psi [-pi pi]/1 -> Product1/1, Interval Test/1, Add1/1
  Interval Test/1 -> Product/1, Logical Operator/1
  Product/1 -> Add/2
  Add/1 -> psi [0 2pi]/1
  Logical Operator/1 -> Product1/2
  angle1/1 -> Add1/2
  Add1/1 -> Product/2
  Product1/1 -> Add/1

== system Chapter_4_Section_3_Model/Ship_Model/LOS2/Subsystem1/Enabled Subsystem ==
  note: This condition means that the ship has reached the last way point
  x : Inport
  y : Inport  Port=2
  Enable : EnablePort  PropagateVarSize=During execution
  Add2 : Sum  Inputs=+-
  Add3 : Sum  Inputs=+-
  Constant1 : Constant  Value=length(X_way)
  Constant2 : Constant  Value=length(X_way)-1
  Constant3 : Constant  Value=length(X_way)-1
  Constant4 : Constant  Value=length(X_way)
  Mux : Mux  Inputs=2
  R_convrg : Constant  Value=Last_Pt_Accuracy
  Relational Operator : RelationalOperator  Operator=<  OutDataTypeStr=boolean  RndMeth=Nearest
  Stop Simulation : Stop
  norm : Fcn  Expr=sqrt(u(1)^2+u(2)^2)
  x-way Lookup Table : Lookup  InputValues=INDEX  Table=X_way
  x-way Lookup Table1 : Lookup  InputValues=INDEX  Table=X_way
  y-way Lookup Table : Lookup  InputValues=INDEX  Table=Y_way
  y-way Lookup Table1 : Lookup  InputValues=INDEX  Table=Y_way
  wires:
  norm/1 -> Relational Operator/1
  R_convrg/1 -> Relational Operator/2
  Relational Operator/1 -> Stop Simulation/1
  x-way Lookup Table/1 -> [x_i]
  y-way Lookup Table/1 -> [y_i]
  x-way Lookup Table1/1 -> [x_i1]
  y-way Lookup Table1/1 -> [y_i1]
  Constant2/1 -> x-way Lookup Table/1
  Constant3/1 -> y-way Lookup Table/1
  Constant1/1 -> x-way Lookup Table1/1
  Constant4/1 -> y-way Lookup Table1/1
  [x_i1] -> Add2/2
  [y_i1] -> Add3/2
  Add2/1 -> Mux/1
  Add3/1 -> Mux/2
  Mux/1 -> norm/1
  x/1 -> Add2/1
  y/1 -> Add3/1

== system Chapter_4_Section_3_Model/Ship_Model/LOS2/Subsystem1/Subsystem ==
  note: P
  note: A
  note: B
  note: det(B-A,P-A)
  x : Inport
  y : Inport  Port=2
  x_i : Inport  Port=3
  y_i : Inport  Port=4
  x_i1 : Inport  Port=5
  y_i1 : Inport  Port=6
  Add{1..5} (5 alike) : Sum  Inputs=+-
  Product1 : Product  RndMeth=Zero
  Product2 : Product  RndMeth=Zero
  det : Outport
  wires:
  x/1 -> [x]
  y/1 -> [y]
  x_i/1 -> [x_i]
  y_i/1 -> [y_i]
  x_i1/1 -> [x_i1]
  y_i1/1 -> [y_i1]
  [x_i1] -> Add2/1
  [x_i] -> Add2/2
  [y] -> Add1/1
  [y_i] -> Add1/2
  Add2/1 -> Product2/1
  Add1/1 -> Product2/2
  Product2/1 -> Add3/1
  Add5/1 -> Product1/1
  Add4/1 -> Product1/2
  [x] -> Add5/1
  [x_i] -> Add5/2
  [y_i1] -> Add4/1
  [y_i] -> Add4/2
  Product1/1 -> Add3/2
  Add3/1 -> det/1

== system Chapter_4_Section_3_Model/Ship_Model/LOS2/Subsystem1/Subsystem1 ==
  x_i1 : Inport
  "x_i " : Inport  Port=2
  y_i1 : Inport  Port=3
  y_i : Inport  Port=4
  Add10 : Sum
  Add8 : Sum  Inputs=+-
  Add9 : Sum  Inputs=+-
  Math Function : Math  Operator=square  SaturateOnIntegerOverflow=on
  Math Function1 : Math  Operator=square  SaturateOnIntegerOverflow=on
  Math Function2 : Math  Operator=sqrt  SaturateOnIntegerOverflow=on
  Trigonometric Function : Trigonometry  Operator=atan2
  norm_ : Outport
  slope_waypath : Outport  Port=2
  wires:
  Add8/1 -> Math Function/1, Trigonometric Function/2
  Add9/1 -> Math Function1/1, Trigonometric Function/1
  Math Function/1 -> Add10/1
  Math Function1/1 -> Add10/2
  Add10/1 -> Math Function2/1
  x_i1/1 -> Add8/1
  "x_i "/1 -> Add8/2
  Math Function2/1 -> norm_/1
  y_i1/1 -> Add9/1
  y_i/1 -> Add9/2
  Trigonometric Function/1 -> slope_waypath/1

== system Chapter_4_Section_3_Model/Ship_Model/Ship Dynamics with Environmental Forces and Memory Effect/Buoyancy_Forces/Cross Product ==
  a : Inport
  b : Inport  Port=2
  Demux : Demux  Outputs=3
  Demux1 : Demux  Outputs=3
  Mux : Mux  Inputs=3
  Product{,1..5} (6 alike) : Product  RndMeth=Zero
  Subtract : Sum  Inputs=+-
  Subtract2 : Sum  Inputs=+-
  Subtract3 : Sum  Inputs=+-
  c : Outport
  wires:
  a/1 -> Demux/1
  b/1 -> Demux1/1
  Product/1 -> Subtract/1
  Product2/1 -> Subtract/2
  Demux/2 -> Product/1, Product5/1
  Demux1/3 -> Product/2, Product3/2
  Demux/3 -> Product2/1, Product1/1
  Demux1/2 -> Product2/2, Product4/2
  Demux1/1 -> Product1/2, Product5/2
  Product1/1 -> Subtract2/1
  Demux/1 -> Product3/1, Product4/1
  Product3/1 -> Subtract2/2
  Product4/1 -> Subtract3/1
  Product5/1 -> Subtract3/2
  Subtract/1 -> Mux/1
  Subtract2/1 -> Mux/2
  Subtract3/1 -> Mux/3
  Mux/1 -> c/1

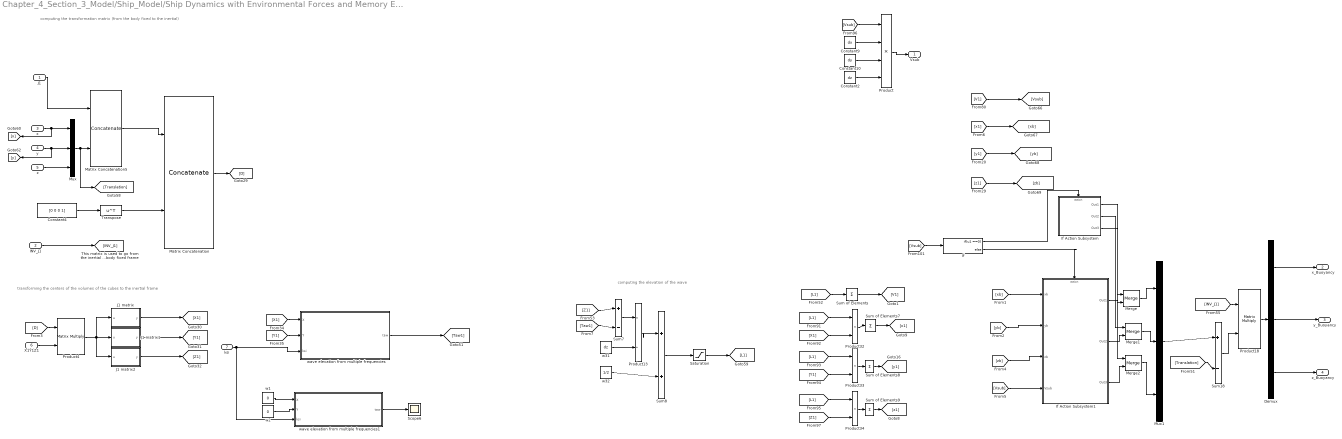
== system Chapter_4_Section_3_Model/Ship_Model/Ship Dynamics with Environmental Forces and Memory Effect/Buoyancy_Forces/Subsystem ==
  note: computing the transformation matrix (from the body fixed to the inertial)
  note: computing the elevation of the wave
  note: transforming the centers of the volumes of the cubes to the inertial frame
  J1 : Inport
  INV_J1 : Inport  Port=2
  x : Inport  Port=3
  y : Inport  Port=4
  z : Inport  Port=5
  X1Y1Z1 : Inport  Port=6
  ksi : Inport  Port=7
  Constant10 : Constant  Value=dy
  Constant2 : Constant  Value=dz
  Constant4 : Constant  Value=[0 0 0 1]
  Constant9 : Constant  Value=dx
  Demux : Demux  Outputs=3
  If : If  IfExpression=u1 ==0
  If Action Subsystem : Subsystem  TreatAsAtomicUnit=on
  If Action Subsystem1 : Subsystem  TreatAsAtomicUnit=on
  J1 matrix : MATLAB Function  TreatAsAtomicUnit=on
  J1 matrix1 : MATLAB Function  TreatAsAtomicUnit=on
  J1 matrix2 : MATLAB Function  TreatAsAtomicUnit=on
  Matrix Concatenation : Concatenate  Mode=Multidimensional array
  Matrix Concatenation5 : Concatenate  Mode=Multidimensional array  ConcatenateDimension=2
  Merge : Merge
  Merge1 : Merge
  Merge2 : Merge
  Mux : Mux  Inputs=3
  Mux1 : Mux  Inputs=3
  Product : Product  Inputs=4  RndMeth=Zero
  Product13 : Product  Inputs=*/  RndMeth=Zero
  Product18 : Product  Multiplication=Matrix(*)  RndMeth=Zero
  Product32 : Product  RndMeth=Zero
  Product33 : Product  RndMeth=Zero
  Product34 : Product  RndMeth=Zero
  Product4 : Product  Multiplication=Matrix(*)  RndMeth=Zero
  Saturation : Saturate  UpperLimit=1  LowerLimit=0
  Scope6 : Scope
  Sum of Elements{,7..9} (4 alike) : Sum  Inputs=+
  Sum18 : Sum  Inputs=|+|-|
  Sum7 : Sum  Inputs=|+|-|
  Sum8 : Sum  Inputs=|+|+|
  Transpose : Math  Operator=transpose  SaturateOnIntegerOverflow=on
  w1 : Constant  Value=0
  w2 : Constant  Value=0
  w31 : Constant  Value=dz
  w32 : Constant  Value=1/2
  wave elevation from multiple frequencies : Subsystem
  wave elevation from multiple frequencies1 : Subsystem
  Vsub : Outport
  x_Buoyancy : Outport  Port=2
  y_Buoyancy : Outport  Port=3
  z_Buoyancy : Outport  Port=4
  wires:
  [Vsub] -> Product/1
  Constant9/1 -> Product/2
  Constant10/1 -> Product/3
  Constant2/1 -> Product/4
  [V1] -> [Vsub]
  Product/1 -> Vsub/1
  [x1] -> [xb]
  [y1] -> [yb]
  [D] -> Product4/1
  X1Y1Z1/1 -> Product4/2
  Mux/1 -> Matrix Concatenation5/2, [Translation]
  J1/1 -> Matrix Concatenation5/1
  x/1 -> Mux/1, [x]
  y/1 -> Mux/2, [y]
  z/1 -> Mux/3
  Constant4/1 -> Transpose/1
  Matrix Concatenation5/1 -> Matrix Concatenation/1
  Transpose/1 -> Matrix Concatenation/2
  Matrix Concatenation/1 -> [D]
  Product4/1 -> J1 matrix2/1(u), J1 matrix1/1(u), J1 matrix/1(u)
  J1 matrix/1(y) -> [X1]
  J1 matrix1/1(y) -> [Y1]
  J1 matrix2/1(y) -> [Z1]
  [Z1] -> Sum7/1
  [Taw1] -> Sum7/2
  Sum7/1 -> Product13/1
  w31/1 -> Product13/2
  Product13/1 -> Sum8/1
  w32/1 -> Sum8/2
  [L1] -> Sum of Elements/1
  Sum of Elements/1 -> [V1]
  [L1] -> Product32/1
  [X1] -> Product32/2
  Product32/1 -> Sum of Elements7/1
  [L1] -> Product33/1
  [Y1] -> Product33/2
  Product33/1 -> Sum of Elements8/1
  [L1] -> Product34/1
  [Z1] -> Product34/2
  Product34/1 -> Sum of Elements9/1
  Sum of Elements7/1 -> [x1]
  Sum of Elements8/1 -> [y1]
  Sum of Elements9/1 -> [z1]
  [z1] -> [zb]
  Mux1/1 -> Sum18/1
  [Translation] -> Sum18/2
  [INV_J1] -> Product18/1
  Sum18/1 -> Product18/2
  Product18/1 -> Demux/1
  Demux/1 -> x_Buoyancy/1
  Demux/2 -> y_Buoyancy/1
  Demux/3 -> z_Buoyancy/1
  INV_J1/1 -> [INV_J1]
  Sum8/1 -> Saturation/1
  Saturation/1 -> [L1]
  [X1] -> wave elevation from multiple frequencies/1(X)
  [Y1] -> wave elevation from multiple frequencies/2(Y)
  wave elevation from multiple frequencies/1(taw) -> [Taw1]
  w1/1 -> wave elevation from multiple frequencies1/1(X)
  w2/1 -> wave elevation from multiple frequencies1/2(Y)
  wave elevation from multiple frequencies1/1(taw) -> Scope6/1
  [Vsub] -> If/1
  [xb] -> If Action Subsystem1/1(xb)
  [yb] -> If Action Subsystem1/2(yb)
  [zb] -> If Action Subsystem1/3(zb)
  [Vsub] -> If Action Subsystem1/4(Vsub)
  If/2 -> If Action Subsystem1/Action
  If/1 -> If Action Subsystem/Action
  If Action Subsystem/1(Out1) -> Merge/1
  If Action Subsystem1/1(Out1) -> Merge/2
  If Action Subsystem/2(Out2) -> Merge1/1
  If Action Subsystem1/2(Out2) -> Merge1/2
  If Action Subsystem/3(Out3) -> Merge2/1
  If Action Subsystem1/3(Out3) -> Merge2/2
  Merge/1 -> Mux1/1
  Merge1/1 -> Mux1/2
  Merge2/1 -> Mux1/3
  ksi/1 -> wave elevation from multiple frequencies/3(ksi), wave elevation from multiple frequencies1/3(ksi)

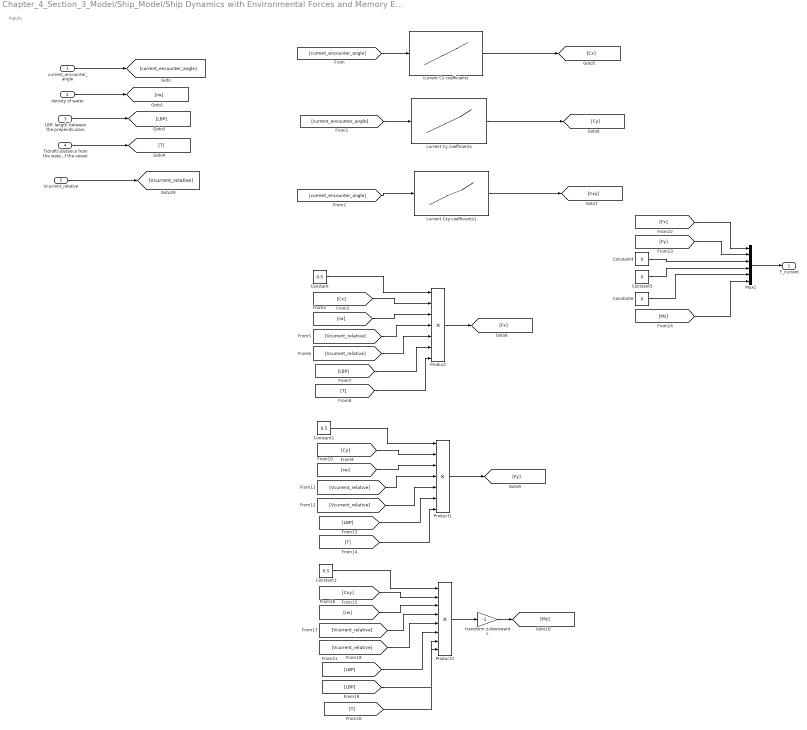
== system Chapter_4_Section_3_Model/Ship_Model/Ship Dynamics with Environmental Forces and Memory Effect/Current Force/Subsystem4 ==
  note: Inputs
  "current_encounter_angle " : Inport
  density of water : Inport  Port=2
  LBP: length between the prependiculars : Inport  Port=3
  "T(draft):distance from the water line to the bottom of the vessel   " : Inport  Port=4
  Vcurrent_relative : Inport  Port=5
  Constant : Constant  Value=0.5
  Constant1 : Constant  Value=0.5
  Constant3 : Constant  Value=0.5
  Constant4 : Constant  Value=0
  Constant5 : Constant  Value=0
  Constant6 : Constant  Value=0
  Mux1 : Mux  Inputs=6
  Product : Product  Inputs=7  RndMeth=Zero
  Product1 : Product  Inputs=7  RndMeth=Zero
  Product3 : Product  Inputs=8  RndMeth=Zero
  current Cx coefficients : Lookup  InputValues="[0    8.2220   15.2263   24.5694   31.5833   38.6069   42.8231   49.3779   54.5194   61.0550   65.2493   70.8402   78.2891 85.7283   90.3720   95.4772   99.1932  104.7744  110.3605  116.4225  120.1602  122.0351  126.7272  132.3591  136.5825  140.3347 142.6735  148.7621  154.3723  160.4464  164.6456  167.9097  172.5752  175.8418  180.0000  184.1582  187.4248  192.0903  195.3544  199.5536  205.6277  211.2379  217.3265  219.6653  223.4175  227.6409  233.2728  237.9649  239.8398  243.5775  249.6395  255.2256  260.8068  264.5228  269.6280  274.2717  281.7109  289.1598  294.7507  298.9450  305.4806  310.6221  317.1769  321.3931  328.4167  335.4306  344.7737  351.7780  360.0000]"  Table="[0.0472    0.0455    0.0419    0.0356    0.0283    0.0172    0.0099   -0.0003   -0.0048   -0.0075   -0.0064   -0.0044    0.0004    0.0090    0.0166    0.0260    0.0317    0.0375    0.0413    0.0415   0.0388    0.0351    0.0240    0.0101   -0.0001   -0.0084   -0.0112   -0.0213   -0.0268   -0.0313   -0.0321   -0.0321   -0.0329   -0.0338   -0.0336   -0.0338   -0.0329   -0.0321   -0.0321   -0.0313  -0.0268   -0.0213   -0.0112   -0.0084   -0.0001    0.0101    0.0240    0.0351    0.0388    0.0415    0.0413    0.0375    0.0317    0.0260    0.0166    0.0090    0.0004   -0.0044   -0.0064   -0.0075   -0.0048   -0.0003    0.0099    0.0172    0.0283    0.0356    0.0419    0.0455    0.0472]"  LookUpMeth=Interpolation-Use End Values  RndMeth=Nearest
  current Cxy coefficients1 : Lookup  InputValues="[0    7.9070   17.2093   26.5116   37.6744   47.4418   58.1395   68.8372   78.6046   86.9767   96.2790  104.1860  113.0232  121.8604  131.1627  141.3953  149.7674  160.4650 169.3022  180.0000  190.6978  199.5350  210.2326  218.6047  228.8373  238.1396  246.9768  255.8140  263.7210  273.0233  281.3954  291.1628  301.8605  312.5582  322.3256  333.4884 342.7907  352.0930  360.0000]"  Table="[0   -0.0281   -0.0512   -0.0673   -0.0788   -0.0810   -0.0715   -0.0574   -0.0387   -0.0223    0.0011    0.0152    0.0316    0.0433    0.0504    0.0506    0.0437    0.0323 0.0184         0   -0.0184   -0.0323   -0.0437   -0.0506   -0.0504   -0.0433   -0.0316   -0.0152   -0.0011    0.0223    0.0387    0.0574    0.0715    0.0810    0.0788    0.0673 0.0512    0.0281         0]"  LookUpMeth=Interpolation-Use End Values  RndMeth=Nearest
  current Cy coefficients : Lookup  InputValues="[ 0    4.6559   11.1723   16.7609   23.7448   31.1950   34.4544   38.1801   45.6291   50.2851   55.4061   61.4586   67.5099   76.3518   83.3309   91.2391   97.7495  104.7225  118.6663  128.4253  134.0018  139.5772  149.7989  158.6252  162.8064  170.7049  175.3525  180.0000  184.6475  189.2951  197.1936  201.3748  210.2011  220.4228  225.9982  231.5747  241.3337  255.2775  262.2505  268.7609  276.6691  283.6482  292.4901  298.5414  304.5939  309.7149  314.3709  321.8199  325.5456  328.8050  336.2552  343.2391  348.8277  355.3441  360.0000]"  Table="[0    0.0198    0.0575    0.1139    0.1703    0.2360    0.2642    0.3018    0.3582    0.3958    0.4334    0.4804    0.5181    0.5559    0.5749    0.5846    0.5756    0.5479   0.4738    0.4088    0.3717    0.3252    0.2416    0.1579    0.1207    0.0557    0.0278         0   -0.0278   -0.0557   -0.1207   -0.1579   -0.2416   -0.3252   -0.3717   -0.4088  -0.4738   -0.5479   -0.5756   -0.5846   -0.5749   -0.5559   -0.5181   -0.4804   -0.4334   -0.3958   -0.3582   -0.3018   -0.2642   -0.2360   -0.1703   -0.1139   -0.0575   -0.0198   0]"  LookUpMeth=Interpolation-Use End Values  RndMeth=Nearest
  transform z-downwards : Gain  Gain=-1
  F_current : Outport
  wires:
  "current_encounter_angle "/1 -> [current_encounter_angle]
  density of water/1 -> [rw]
  LBP: length between the prependiculars/1 -> [LBP]
  "T(draft):distance from the water line to the bottom of the vessel   "/1 -> [T]
  [current_encounter_angle] -> current Cx coefficients/1
  [current_encounter_angle] -> current Cy coefficients/1
  [current_encounter_angle] -> current Cxy coefficients1/1
  Constant/1 -> Product/1
  [Cx] -> Product/2
  [rw] -> Product/3
  [Vcurrent_relative] -> Product/4
  [Vcurrent_relative] -> Product/5
  [LBP] -> Product/6
  [T] -> Product/7
  Product/1 -> [Fx]
  Constant1/1 -> Product1/1
  [Cy] -> Product1/2
  [rw] -> Product1/3
  [LBP] -> Product1/6
  [T] -> Product1/7
  Product1/1 -> [Fy]
  Constant3/1 -> Product3/1
  [Cxy] -> Product3/2
  [rw] -> Product3/3
  [Vcurrent_relative] -> Product3/4
  [Vcurrent_relative] -> Product3/5
  [LBP] -> Product3/6
  [LBP] -> Product3/7
  Product3/1 -> transform z-downwards/1
  [T] -> Product3/8
  Vcurrent_relative/1 -> [Vcurrent_relative]
  [Vcurrent_relative] -> Product1/4
  [Vcurrent_relative] -> Product1/5
  transform z-downwards/1 -> [Mz]
  Mux1/1 -> F_current/1
  [Fx] -> Mux1/1
  [Fy] -> Mux1/2
  Constant4/1 -> Mux1/3
  Constant5/1 -> Mux1/4
  Constant6/1 -> Mux1/5
  [Mz] -> Mux1/6
  current Cx coefficients/1 -> [Cx]
  current Cy coefficients/1 -> [Cy]
  current Cxy coefficients1/1 -> [Cxy]
